simulink model "ballonbeam_matlab1"  (R2025b)
settings: Solver=VariableStepAuto  StartTime=0.0  StopTime=10.0  RelTol=1e-3
values from neighbouring files (symbols this model uses):
  K1 = K2    (= 11.67)    [par_regulatora_APRBS.m]    (also in parametry_reg.m = mean(K_obl))
  K2 = 11.67    [par_regulatora_APRBS.m]
  Kp = 1    [identyfikacja_skok.m]    (also in par_regulatora_APRBS.m = 0.13888689828; parametry_reg.m = wn1^(2)/K1)
  Td = 1    [identyfikacja_skok.m]    (also in par_regulatora_APRBS.m = 0.0705035052842; parametry_reg.m = (2*ksi*wn1)/K1)
  Ti = 1    [identyfikacja_skok.m]    (also in parametry_reg.m = 3)
  To = 0.3    [par_regulatora_APRBS.m]
  Ts = 0.03    [dane_wymuszenia.mat]    (also in generowanie_APRBS1.m; par_regulatora_APRBS.m = 0.6766; wczytanie_identyfikacji.m = 0.034)
settings Model: Creator=mati  LastModifiedBy=mati

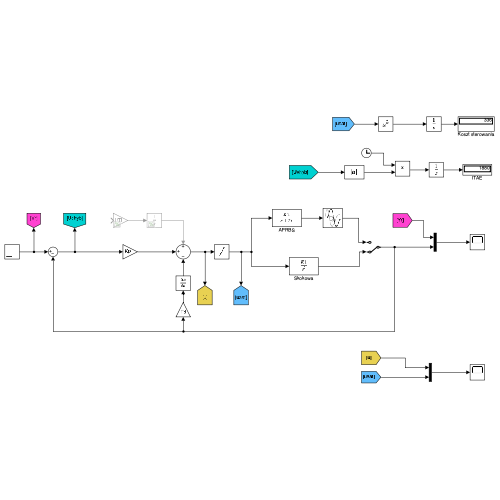
[thumbnail: Simulink's stored preview of the top-level diagram]
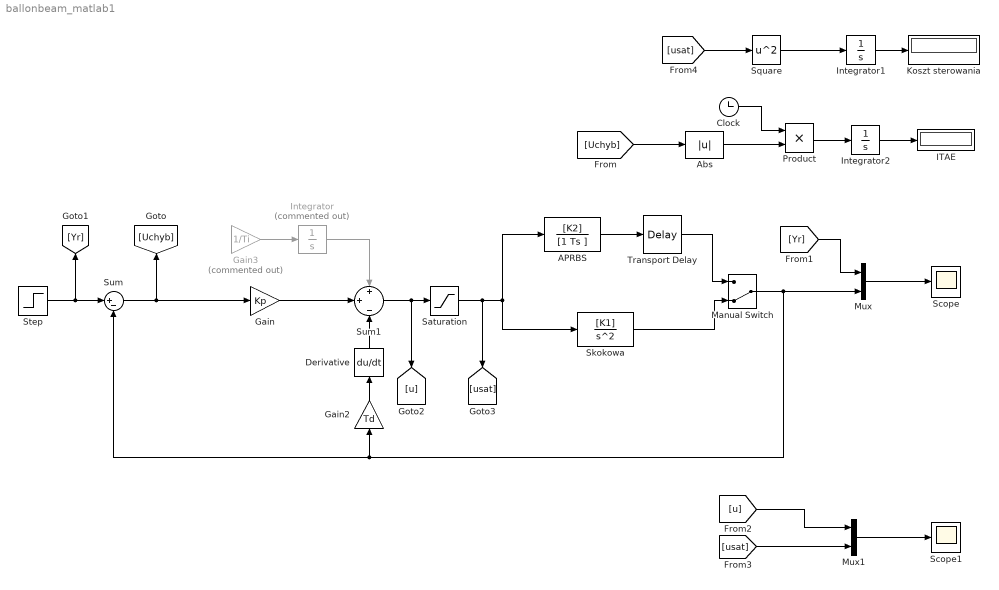
== system ballonbeam_matlab1 ==
  APRBS : TransferFcn  Numerator=[K2]  Denominator=[1 Ts ]
  Abs : Abs  SaturateOnIntegerOverflow=off
  Clock : Clock
  Derivative : Derivative
  Gain : Gain  Gain=Kp
  Gain2 : Gain  Gain=Td
  Gain3 : Gain  Commented=on  Gain=1/Ti
  ITAE : Display
  Integrator : Integrator  Commented=on
  Integrator1 : Integrator
  Integrator2 : Integrator
  Koszt sterowania : Display
  Manual Switch : ManualSwitch  CurrentSetting=0
  Mux : Mux  Inputs=2
  Mux1 : Mux  Inputs=2
  Product : Product
  Saturation : Saturate  UpperLimit=30  LowerLimit=-30
  Scope : Scope
      settings: ActiveDisplayYMinimum=-15.284496038986166  ActiveDisplayYMaximum=137.56046435087552
  Scope1 : Scope
  Skokowa : TransferFcn  Numerator=[K1]  Denominator=[1 0 0]
  Square : Math  Operator=square
  Step : Step  After=120  SampleTime=0
  Sum : Sum  Inputs=|+-
  Sum1 : Sum  Inputs=+|+|-
  Transport Delay : TransportDelay  DelayTime=To
  wires:
  Gain/1 -> Sum1/2
  Sum/1 -> Gain/1, [Uchyb]
  Skokowa/1 -> Manual Switch/2
  Manual Switch/1 -> Sum/2, Gain2/1, Mux/2
  APRBS/1 -> Transport Delay/1
  Gain3/1 -> Integrator/1
  Gain2/1 -> Derivative/1
  Derivative/1 -> Sum1/3
  Sum1/1 -> [u], Saturation/1
  Saturation/1 -> [usat], APRBS/1, Skokowa/1
  Step/1 -> Sum/1, [Yr]
  Mux/1 -> Scope/1
  [Yr] -> Mux/1
  [usat] -> Mux1/2
  [u] -> Mux1/1
  Mux1/1 -> Scope1/1
  Abs/1 -> Product/2
  Clock/1 -> Product/1
  [Uchyb] -> Abs/1
  Product/1 -> Integrator2/1
  Integrator2/1 -> ITAE/1
  Square/1 -> Integrator1/1
  Integrator1/1 -> Koszt sterowania/1
  [usat] -> Square/1
  Integrator/1 -> Sum1/1
  Transport Delay/1 -> Manual Switch/1
